simulink model "SolarPanelModel"  (R2023a)
settings: Solver=VariableStepAuto  StartTime=0.0  StopTime=10.0  RelTol=1e-3
undefined symbols (not defined in the file or in its folder): Acid, Lead
libraries: spsSeriesRLCBranchLib x6, spsBatteryLib x2, spsDiodeLib x2, spsMosfetLib x2, simulink x2, spsPVArrayLib x2, spsVoltageMeasurementLib x2, spspowerguiLib x2
settings Model: Creator=Vivek Rajput  LastModifiedBy=Vivek Rajput

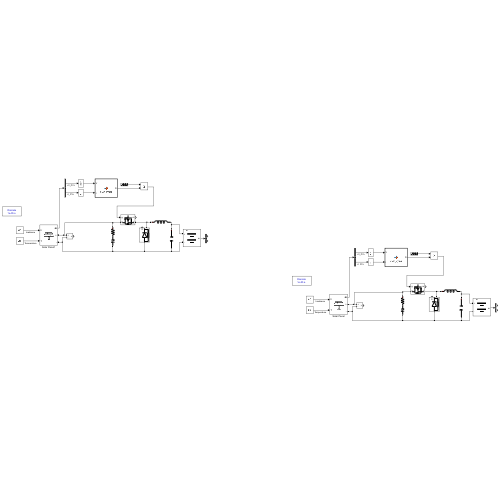
[thumbnail: Simulink's stored preview of the top-level diagram]
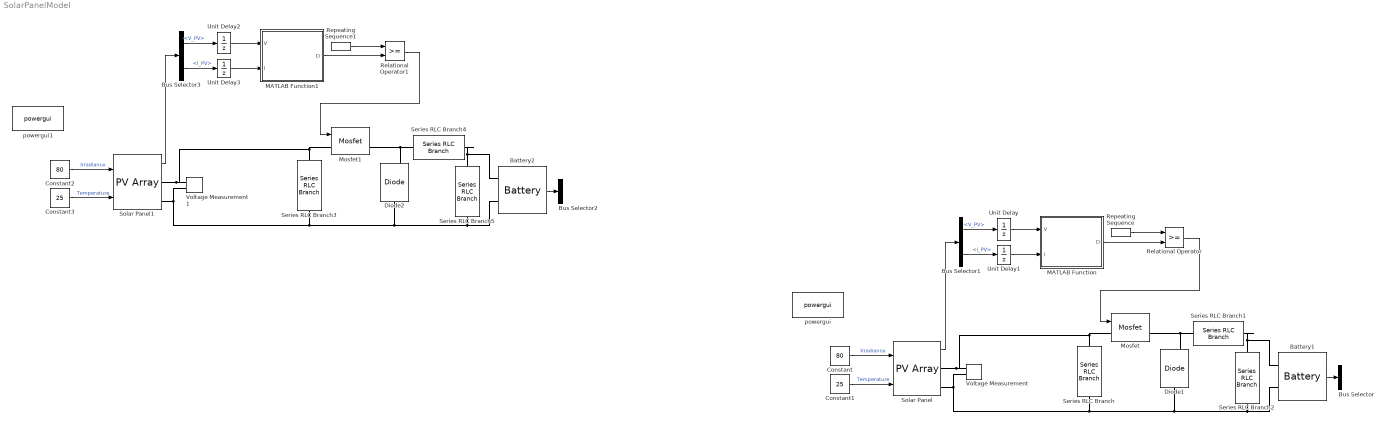
== system SolarPanelModel ==
  Battery1 : spsBatteryLib/Battery  BatType=Lead-Acid  ShowTempParam=off  ThermalPreset=no  ShowAgeParam=off  NomV=12  NomQ=100  SOC=45  Batt_Tr=1  PresetModel=on  MaxQ=104.1667  MinV=9  FullV=13.0658  Dis_rate=20  R=0.0012  Normal_OP=31.0278  expZone="[12.2171     0.333333]"  current=[6.5 13 32.5]  Units=Time  Tci=20  NomT=20  T2=-30  MaxQ2=4.8  FullV2=7.1  Normal_OP2=5.655  expZone2="[6.58           1]"  Rca=0.6  ti=2000  Dp=0  Neq0=0  Tsim=1e6  Ta1=25  Qeol=5.4*0.9  Reol=0.013333*1.2  Char_age=[2.3478, 3]  Dis_age=[2.3478, 10]  N1=1500  N2=10500  N3=1000  N4=1400  Ta2=45  N5=950
  Battery2 : spsBatteryLib/Battery  BatType=Lead-Acid  ShowTempParam=off  ThermalPreset=no  ShowAgeParam=off  NomV=12  NomQ=100  SOC=45  Batt_Tr=1  PresetModel=on  MaxQ=104.1667  MinV=9  FullV=13.0658  Dis_rate=20  R=0.0012  Normal_OP=31.0278  expZone="[12.2171     0.333333]"  current=[6.5 13 32.5]  Units=Time  Tci=20  NomT=20  T2=-30  MaxQ2=4.8  FullV2=7.1  Normal_OP2=5.655  expZone2="[6.58           1]"  Rca=0.6  ti=2000  Dp=0  Neq0=0  Tsim=1e6  Ta1=25  Qeol=5.4*0.9  Reol=0.013333*1.2  Char_age=[2.3478, 3]  Dis_age=[2.3478, 10]  N1=1500  N2=10500  N3=1000  N4=1400  Ta2=45  N5=950
  Bus Selector : BusSelector  OutputSignals=Current (A),Voltage (V)
  Bus Selector1 : BusSelector  OutputSignals=V_PV,I_PV
  Bus Selector2 : BusSelector  OutputSignals=Current (A),Voltage (V)
  Bus Selector3 : BusSelector  OutputSignals=V_PV,I_PV
  Constant : Constant  Value=80
  Constant1 : Constant  Value=25
  Constant2 : Constant  Value=80
  Constant3 : Constant  Value=25
  Diode1 : spsDiodeLib/Diode  Ron=0.001  Lon=0  Vf=0.8  IC=0  UseSnubber=0  Rs=500  Cs=250e-9  Measurements=on
  Diode2 : spsDiodeLib/Diode  Ron=0.001  Lon=0  Vf=0.8  IC=0  UseSnubber=0  Rs=500  Cs=250e-9  Measurements=on
  MATLAB Function : MATLAB Function  TreatAsAtomicUnit=on
  MATLAB Function1 : MATLAB Function  TreatAsAtomicUnit=on
  Mosfet : spsMosfetLib/Mosfet  Ron=0.1  Lon=0  Rd=0.01  Vfd=0  IC=0  Rs=1e5  Cs=inf  Measurements=on
  Mosfet1 : spsMosfetLib/Mosfet  Ron=0.1  Lon=0  Rd=0.01  Vfd=0  IC=0  Rs=1e5  Cs=inf  Measurements=on
  Relational Operator : RelationalOperator  OutDataTypeStr=boolean  RndMeth=Simplest  InputSameDT=off
  Relational Operator1 : RelationalOperator  OutDataTypeStr=boolean  RndMeth=Simplest  InputSameDT=off
  Repeating Sequence : simulink/Sources/Repeating Sequence  rep_seq_t=[0 0.0002]  rep_seq_y=[0 1]
  Repeating Sequence1 : simulink/Sources/Repeating Sequence  rep_seq_t=[0 0.0002]  rep_seq_y=[0 1]
  Series RLC Branch : spsSeriesRLCBranchLib/Series RLC Branch  LConnTagsString=__new0  RConnTagsString=__new0  BranchType=RC  Resistance=0.001  Inductance=1e-3  SetiL0=off  InitialCurrent=0  Capacitance=10000e-6  Setx0=off  InitialVoltage=0  Measurements=None
  Series RLC Branch1 : spsSeriesRLCBranchLib/Series RLC Branch  LConnTagsString=__new0  RConnTagsString=__new0  BranchType=L  Resistance=0.001  Inductance=0.8653e-3  SetiL0=off  InitialCurrent=0  Capacitance=10000e-6  Setx0=off  InitialVoltage=0  Measurements=None
  Series RLC Branch2 : spsSeriesRLCBranchLib/Series RLC Branch  LConnTagsString=__new0  RConnTagsString=__new0  BranchType=C  Resistance=0.001  Inductance=0.8653e-3  SetiL0=off  InitialCurrent=0  Capacitance=369.79e-6  Setx0=off  InitialVoltage=0  Measurements=None
  Series RLC Branch3 : spsSeriesRLCBranchLib/Series RLC Branch  LConnTagsString=__new0  RConnTagsString=__new0  BranchType=RC  Resistance=0.001  Inductance=1e-3  SetiL0=off  InitialCurrent=0  Capacitance=10000e-6  Setx0=off  InitialVoltage=0  Measurements=None
  Series RLC Branch4 : spsSeriesRLCBranchLib/Series RLC Branch  LConnTagsString=__new0  RConnTagsString=__new0  BranchType=L  Resistance=0.001  Inductance=0.8653e-3  SetiL0=off  InitialCurrent=0  Capacitance=10000e-6  Setx0=off  InitialVoltage=0  Measurements=None
  Series RLC Branch5 : spsSeriesRLCBranchLib/Series RLC Branch  LConnTagsString=__new0  RConnTagsString=__new0  BranchType=C  Resistance=0.001  Inductance=0.8653e-3  SetiL0=off  InitialCurrent=0  Capacitance=369.79e-6  Setx0=off  InitialVoltage=0  Measurements=None
  Solar Panel : spsPVArrayLib/PV Array  Npar=40  Nser=10  PlotType=array @ 25 deg.C & specified irradiances  S_vec="[ 1000  500  100 ]"  Temp_C_vec="[ 45 25  ]"  ModuleName=User-defined  PlotWhenSelected=off  Pm=213.15  Ncell=60  Voc=36.3  Isc=7.84  Vm=29  Im=7.35  beta_Voc_pc=-0.36099  alpha_Isc_pc=0.102  beta_Voc=-0.13104  alpha_Isc=0.0079968  IL=7.8654  I0=2.9273e-10  nI=0.98119  Rsh=313.0553  Rs=0.39381  RobustModel=off  RobustCellTemperature=313.3991  BAL=on  Tc=1e-6  Tfilter=5e-5
  Solar Panel1 : spsPVArrayLib/PV Array  Npar=40  Nser=10  PlotType=array @ 25 deg.C & specified irradiances  S_vec="[ 1000  500  100 ]"  Temp_C_vec="[ 45 25  ]"  ModuleName=User-defined  PlotWhenSelected=off  Pm=213.15  Ncell=60  Voc=36.3  Isc=7.84  Vm=29  Im=7.35  beta_Voc_pc=-0.36099  alpha_Isc_pc=0.102  beta_Voc=-0.13104  alpha_Isc=0.0079968  IL=7.8654  I0=2.9273e-10  nI=0.98119  Rsh=313.0553  Rs=0.39381  RobustModel=off  RobustCellTemperature=313.3991  BAL=on  Tc=1e-6  Tfilter=5e-5
  Unit Delay{,1..3} (4 alike) : UnitDelay  SampleTime=1e-4  HasFrameUpgradeWarning=on
  Voltage Measurement : spsVoltageMeasurementLib/Voltage Measurement  PhasorSimulation=off  OutputType=Complex  PSBequivalent=0
  Voltage Measurement1 : spsVoltageMeasurementLib/Voltage Measurement  PhasorSimulation=off  OutputType=Complex  PSBequivalent=0
  powergui : spspowerguiLib/powergui  Priority=1  SimulationMode=Discrete  SampleTime=10e-6  frequency=60  Iterations=50  frequencyindice=0  Pbase=100e6  ErrMax=1e-4  UnitsV=kV  UnitsW=MW  buscounter=0  FunctionMessages=off  echomessages=off  EnableUseOfTLC=off  CurrentSourceSwitches=off  DisableSnubberDevices=off  DisableRonSwitches=off  DisableVfSwitches=off  DisplayEquations=off  AutomaticDiscreteSolvers=off  SolverType=Tustin/Backward Euler (TBE)  Interpol=off  ExternalGateDelay=off  methode=off  Ts=100  x0status=blocks  SPID=on  SwTol=0  HookPort=off  NonlinearTolerance=1e-4  nMaxIteration=100  ContinueOnMaxIteration=off  RestoreLinks=warning  ResistiveCurrentMeasurement=off  Frange=[0:2:500]  Ylog=off  Xlog=on  ShowGrid=off  save=off  variable=ZData  structure=0  ZoomFFT=off  StartTime=0.0  cycles=1  DisplayStyle=1  fundamental=60  FreqAxis=off  MaxFrequency=1000  frequencyindicesteady=1  RmsSteady=1  display=off
  powergui1 : spspowerguiLib/powergui  Priority=1  SimulationMode=Discrete  SampleTime=10e-6  frequency=60  Iterations=50  frequencyindice=0  Pbase=100e6  ErrMax=1e-4  UnitsV=kV  UnitsW=MW  buscounter=0  FunctionMessages=off  echomessages=off  EnableUseOfTLC=off  CurrentSourceSwitches=off  DisableSnubberDevices=off  DisableRonSwitches=off  DisableVfSwitches=off  DisplayEquations=off  AutomaticDiscreteSolvers=off  SolverType=Tustin/Backward Euler (TBE)  Interpol=off  ExternalGateDelay=off  methode=off  Ts=100  x0status=blocks  SPID=on  SwTol=0  HookPort=off  NonlinearTolerance=1e-4  nMaxIteration=100  ContinueOnMaxIteration=off  RestoreLinks=warning  ResistiveCurrentMeasurement=off  Frange=[0:2:500]  Ylog=off  Xlog=on  ShowGrid=off  save=off  variable=ZData  structure=0  ZoomFFT=off  StartTime=0.0  cycles=1  DisplayStyle=1  fundamental=60  FreqAxis=off  MaxFrequency=1000  frequencyindicesteady=1  RmsSteady=1  display=off
  wires:
  Constant/1 -> Solar Panel/1  "Irradiance"
  Constant1/1 -> Solar Panel/2  "Temperature"
  Battery1/1 -> Bus Selector/1
  Solar Panel/1 -> Bus Selector1/1
  Bus Selector1/1 -> Unit Delay/1  "<V_PV>"
  Bus Selector1/2 -> Unit Delay1/1  "<I_PV>"
  Unit Delay/1 -> MATLAB Function/1(V)
  Unit Delay1/1 -> MATLAB Function/2(I)
  MATLAB Function/1(D) -> Relational Operator/2
  Repeating Sequence/1 -> Relational Operator/1
  Relational Operator/1 -> Mosfet/1
  Constant3/1 -> Solar Panel1/2  "Temperature"
  Repeating Sequence1/1 -> Relational Operator1/1
  Relational Operator1/1 -> Mosfet1/1
  Solar Panel1/1 -> Bus Selector3/1
  Unit Delay3/1 -> MATLAB Function1/2(I)
  Battery2/1 -> Bus Selector2/1
  Unit Delay2/1 -> MATLAB Function1/1(V)
  Bus Selector3/2 -> Unit Delay3/1  "<I_PV>"
  MATLAB Function1/1(D) -> Relational Operator1/2
  Bus Selector3/1 -> Unit Delay2/1  "<V_PV>"
  Constant2/1 -> Solar Panel1/1  "Irradiance"
  connections:
  Solar Panel/RConn2 -- Battery1/LConn2 -- Series RLC Branch2/RConn1 -- Diode1/LConn1 -- Series RLC Branch/RConn1 -- Voltage Measurement/LConn2
  Solar Panel/RConn1 -- Mosfet/LConn1 -- Series RLC Branch/LConn1 -- Voltage Measurement/LConn1
  Mosfet/RConn1 -- Series RLC Branch1/LConn1 -- Diode1/RConn1
  Series RLC Branch1/RConn1 -- Battery1/LConn1 -- Series RLC Branch2/LConn1
  Series RLC Branch3/LConn1 -- Solar Panel1/RConn1 -- Voltage Measurement1/LConn1 -- Mosfet1/LConn1
  Series RLC Branch5/RConn1 -- Solar Panel1/RConn2 -- Voltage Measurement1/LConn2 -- Series RLC Branch3/RConn1 -- Diode2/LConn1 -- Battery2/LConn2
  Diode2/RConn1 -- Mosfet1/RConn1 -- Series RLC Branch4/LConn1
  Series RLC Branch5/LConn1 -- Series RLC Branch4/RConn1 -- Battery2/LConn1

== matlab function SolarPanelModel/MATLAB Function1 ==
  data: V input; D output; I input
function D = duty_cycle(V, I)
%#codegen
% MPPT Controller using Perturb and Observe (P&O) Algorithm

persistent V_prev I_prev P_prev D_prev;
if isempty(V_prev)
    % Initialize persistent variables
    V_prev = 0;
    I_prev = 0;
    P_prev = 0;
    D_prev = 0.5; % Initial duty cycle (50%)
end

% Calculate current power
P = V * I;

% Define step size for duty cycle adjustment
D_step = 0.01; % Small step for adjusting duty cycle

% Perturb and Observe (P&O) Algorithm
if P > P_prev
    if V > V_prev
        D = D_prev + D_step; % Increase duty cycle
    else
        D = D_prev - D_step; % Decrease duty cycle
    end
else
    if V > V_prev
        D = D_prev - D_step; % Decrease duty cycle
    else
        D = D_prev + D_step; % Increase duty cycle
    end
end

% Limit duty cycle between 0 and 1
D = max(0, min(1, D));

% Update previous values
V_prev = V;
I_prev = I;
P_prev = P;
D_prev = D;

== matlab function SolarPanelModel/MATLAB Function ==
  data: V input; D output; I input
function D = duty_cycle(V, I)
%#codegen
% MPPT Controller using Perturb and Observe (P&O) Algorithm

persistent V_prev I_prev P_prev D_prev;
if isempty(V_prev)
    % Initialize persistent variables
    V_prev = 0;
    I_prev = 0;
    P_prev = 0;
    D_prev = 0.5; % Initial duty cycle (50%)
end

% Calculate current power
P = V * I;

% Define step size for duty cycle adjustment
D_step = 0.01; % Small step for adjusting duty cycle

% Perturb and Observe (P&O) Algorithm
if P > P_prev
    if V > V_prev
        D = D_prev + D_step; % Increase duty cycle
    else
        D = D_prev - D_step; % Decrease duty cycle
    end
else
    if V > V_prev
        D = D_prev - D_step; % Decrease duty cycle
    else
        D = D_prev + D_step; % Increase duty cycle
    end
end

% Limit duty cycle between 0 and 1
D = max(0, min(1, D));

% Update previous values
V_prev = V;
I_prev = I;
P_prev = P;
D_prev = D;
